simulink model "SMDoubleLinkSYM"  (Simulink 8.2)
settings: Solver=ode45  StartTime=0.0  StopTime=10.0  RelTol=1e-3
undefined symbols (not defined in the file or in its folder): BICEP_L, FOREARM_L
settings Model: Creator=Guillermo  LastModifiedBy=Guillermo
settings DataIOCC: SignalLoggingSaveFormat=Dataset
settings OptimizationCC: ExpressionDepthLimit=128
settings DebuggingCC: FcnCallInpInsideContextMsg=EnableAllAsError  StateNameClashWarn=none
settings GRTTargetCC: CombineOutputUpdateFcns=on  GRTInterface=off

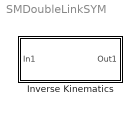
== system SMDoubleLinkSYM ==
  Inverse Kinematics : Subsystem

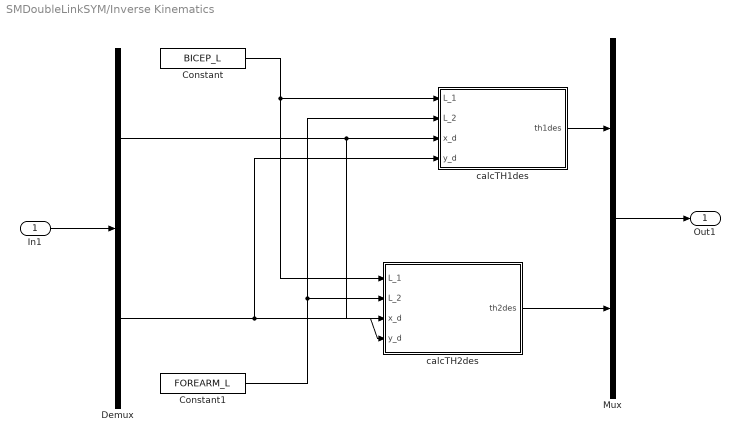
== system SMDoubleLinkSYM/Inverse Kinematics ==
  In1 : Inport
  " calcTH1des" : MATLAB Function  TreatAsAtomicUnit=on
  Constant : Constant  Value=BICEP_L
  Constant1 : Constant  Value=FOREARM_L
  Demux : Demux  Outputs=2
  Mux : Mux  Inputs=2
  calcTH2des : MATLAB Function  TreatAsAtomicUnit=on
  Out1 : Outport
  wires:
  Constant/1 -> calcTH2des/1(L_1), " calcTH1des"/1(L_1)
  Constant1/1 -> " calcTH1des"/2(L_2), calcTH2des/2(L_2)
  Mux/1 -> Out1/1
  calcTH2des/1(th2des) -> Mux/2
  " calcTH1des"/1(th1des) -> Mux/1
  In1/1 -> Demux/1
  Demux/1 -> " calcTH1des"/3(x_d), calcTH2des/3(x_d)
  Demux/2 -> " calcTH1des"/4(y_d), calcTH2des/4(y_d)

== matlab function Inverse Kinematics/calcTH2des ==
  data: L_1 input double; th2des output double; L_2 input double; x_d input double; y_d input double
function th2des = calcTH2des(L_1,L_2,x_d,y_d)
%#codegen

th2des = pi-acos((L_1.^2.*(1.0./2.0)+L_2.^2.*(1.0./2.0)-x_d.^2.*(1.0./2.0)-y_d.^2.));

== matlab function Inverse Kinematics/ calcTH1des ==
  data: L_1 input double; th1des output double; L_2 input double; x_d input double; y_d input double
function th1des = calcTH1des(L_1,L_2,x_d,y_d)
%#codegen

th1des = pi-acos((L_1.^2.*(1.0./2.0)+L_2.^2.*(1.0./2.0)-x_d.^2.*(1.0./2.0)-y_d.^2.));
